simulink model "mcb_pmsm_foc_sensorless_dyno_f28379d"  (R2024b)
settings: Solver=FixedStepDiscrete  StartTime=0.0  StopTime=6  RelTol=1e-3  EnableMultiTasking=on
InitFcn:
  | mcb_pmsm_foc_sensorless_dyno_f28379d_datascript;
model workspace (MAT data in the model file):
  encoderResolution = 2000
  hallOffset = '0.5'
  indexOffset = 850
  polePairs = '4'
undefined symbols (not defined in the file or in its folder): acceleration, dataType, Down, GPTRIP1SEL, GPTRIP2SEL, inverter_motor1, inverter_motor2, PI_params_motor1, PI_params_motor2, pmsm_motor1, pmsm_motor2, PU_System_motor1, PU_System_motor2, PWM_frequency, SlidFCS_params, Speed_openLoop_PU, T_Ref_openLoop, target, Ts, Ts_motor, Ts_simulink, Ts_speed, TZ1, TZ2, Up, Vd_Ref_openLoop_PU
libraries: mcbcontrolslib x20, c2802xlib x14, simulink x8, c280xlib x7, slpidlib x5, c2837xDlib x5, mcbpositiondecoderlib x4, svdschedulerlib x3, mcbsensorlessestimatorlib x2, mcbpmsmnonlinearlib x2, autolibpmsmexterior x2, mcbplantlib x2
(part 4 of 4)

== system mcb_pmsm_foc_sensorless_dyno_f28379d/FOC Algorithm Motor 2/Enable Motor2 after a delay/Delay to start motor2 (codegen)/Disable EnMtr2TrqCtrl ==
  Enable : EnablePort  StatesWhenEnabling=reset
  Constant : Constant  Value=0  OutDataTypeStr=boolean
  Data Store Write : DataStoreWrite  DataStoreName=EnMtr2TrqCtrl  IndexOptions=Index vector (dialog)  Indices=1  OutputSizes=1
  wires:
  Constant/1 -> Data Store Write/1

== system mcb_pmsm_foc_sensorless_dyno_f28379d/FOC Algorithm Motor 2/Enable Motor2 after a delay/Delay to start motor2 (codegen)/Enable EnMtr2TrqCtrl after 2 sec delay ==
  Enable : EnablePort  StatesWhenEnabling=reset
  Add : Sum
  Constant : Constant  OutDataTypeStr=boolean
  Constant1 : Constant  Value=0  OutDataTypeStr=boolean
  Constant2 : Constant  OutDataTypeStr=uint32
  Enable EnMtr2TrqCtrl : Subsystem  TreatAsAtomicUnit=on
  Switch : Switch  Criteria=u2 > Threshold  Threshold=2*PWM_frequency  SaturateOnIntegerOverflow=off  InputSameDT=off
  Unit Delay : UnitDelay  SampleTime=-1  HasFrameUpgradeWarning=on
  wires:
  Constant1/1 -> Switch/3
  Constant/1 -> Switch/1
  Constant2/1 -> Add/1
  Add/1 -> Unit Delay/1, Switch/2
  Unit Delay/1 -> Add/2
  Switch/1 -> Enable EnMtr2TrqCtrl/Enable

== system mcb_pmsm_foc_sensorless_dyno_f28379d/FOC Algorithm Motor 2/Enable Motor2 after a delay/Delay to start motor2 (sim)/Delay 0.5 sec ==
  Enable : EnablePort  StatesWhenEnabling=reset
  Add : Sum
  Constant : Constant  OutDataTypeStr=boolean
  Constant1 : Constant  Value=0  OutDataTypeStr=boolean
  Constant2 : Constant  OutDataTypeStr=uint32
  Switch : Switch  Criteria=u2 > Threshold  Threshold=PWM_frequency/2  SaturateOnIntegerOverflow=off  InputSameDT=off
  Unit Delay : UnitDelay  SampleTime=-1  HasFrameUpgradeWarning=on
  Out1 : Outport
  wires:
  Constant1/1 -> Switch/3
  Constant/1 -> Switch/1
  Constant2/1 -> Add/1
  Add/1 -> Unit Delay/1, Switch/2
  Unit Delay/1 -> Add/2
  Switch/1 -> Out1/1

== system mcb_pmsm_foc_sensorless_dyno_f28379d/FOC Algorithm Motor 2/Enable Motor2 after a delay/Delay to start motor2 (sim)/Enabled Subsystem ==
  Enable : EnablePort
  Constant : Constant  OutDataTypeStr=boolean
  Data Store Write : DataStoreWrite  DataStoreName=EnMtr2TrqCtrl  IndexOptions=Index vector (dialog)  Indices=1  OutputSizes=1
  wires:
  Constant/1 -> Data Store Write/1

== system mcb_pmsm_foc_sensorless_dyno_f28379d/FOC Algorithm Motor 2/Enable Motor2 after a delay/Delay to start motor2 (sim)/Enabled Subsystem2 ==
  Enable : EnablePort
  Constant : Constant  Value=0  OutDataTypeStr=boolean
  Data Store Write : DataStoreWrite  DataStoreName=EnMtr2TrqCtrl  IndexOptions=Index vector (dialog)  Indices=1  OutputSizes=1
  wires:
  Constant/1 -> Data Store Write/1

== system mcb_pmsm_foc_sensorless_dyno_f28379d/FOC Algorithm Motor 2/Input Scaling/Calculate Phase Currents/Data_Type ==
  In1 : Inport
  Data_Type_Fixed_Point : Subsystem  VariantControl=~isequal(dataType,'single')
  Data_Type_Float : Subsystem  VariantControl=isequal(dataType,'single')
  Iab_meas_PU : Outport

== system mcb_pmsm_foc_sensorless_dyno_f28379d/FOC Algorithm Motor 2/Input Scaling/Calculate position and speed/Flux Observer ==
  InputSignals : Inport
  Action Port : ActionPort  ActionPortLabel=case [ 1 ]:
  DC component removal : Subsystem
  Data Store Read1 : DataStoreRead  DataStoreName=Enable  IndexOptions=Index vector (dialog)  Indices=1  OutputSizes=1
  Demux2 : Demux
  Flux Observer : mcbpositiondecoderlib/Flux Observer  MotorSelection=PMSM  DataTypeSelect=off  BlockInputUnit=Per-unit  PerUnitVoltage=PU_System_motor2.V_base  PerUnitCurrent=PU_System_motor2.I_base  PositionSelect=on  FluxSelect=off  TorqueSelect=off  PolePairs=4  StatorResistance=pmsm_motor2.Rs  StatorDAxisInductance=pmsm_motor2.Ld  StatorLeakageInductance=0.0068  RotorLeakageInductance=0.0068  MagnetizingInductance=0.0300  CutoffFreq=3.1863  BlockSampleTime=Ts  ParameterBusInput=off  PositionUnit=Per-unit  PositionDatatype=dataType  FluxUnit=Weber  PerUnitFlux=0.1  FluxDatatype=single  TorqueUnit=Nm  PerUnitTorque=100  TorqueDatatype=single  DataType=0
  IIR Filter : mcbcontrolslib/IIR Filter  VariantControl=Low Pass Filter  VariantSelect=Low-pass  FilterConstantInputType=Specify via dialog  Filter_constant=0.01  advancedSettings=off  Ts=50e-6  cutOff_freq=32.1525
  Logical Operator : Logic  Operator=NOT  IconShape=distinctive  AllPortsSameDT=off  OutDataTypeStr=boolean
  Mux2 : Mux  Inputs=2
  Speed Measurement : mcbpositiondecoderlib/Speed Measurement  PositionUnit=Per unit  PositionScalingDatatype=uint32  SpeedCalculationMode=Time interval for speed calculation  SampleTimeAsync=Ts  MaximumApplicationSpeed=60000  SpeedResolution=5e-6  DelayLength=10  MaximumMeasurableSpeed=59999  MeasurableSpeedResolution=2.794e-05  SpeedUnit=Per unit based on dialog  PerUnitSpeed=PU_System_motor2.N_base  SpeedDataType=dataType
  elect2mech : Gain  Gain=1/pmsm_motor2.p  RndMeth=Simplest  OutDataTypeStr=Inherit: Same as input
  Position/Speed : Outport
  wires:
  InputSignals/1 -> DC component removal/1(SigIN)
  Demux2/1 -> Flux Observer/1
  Demux2/2 -> Flux Observer/2
  Mux2/1 -> Position/Speed/1
  Speed Measurement/1 -> IIR Filter/1
  elect2mech/1 -> Mux2/2
  Demux2/3 -> Flux Observer/3  "Ialpha"
  Demux2/4 -> Flux Observer/4  "Ibeta"
  IIR Filter/1 -> elect2mech/1
  Flux Observer/1 -> Mux2/1, Speed Measurement/1
  Logical Operator/1 -> Flux Observer/5
  Data Store Read1/1 -> Logical Operator/1
  DC component removal/1(SigOUT) -> Demux2/1

== system mcb_pmsm_foc_sensorless_dyno_f28379d/FOC Algorithm Motor 2/Input Scaling/Calculate position and speed/Sliding Mode Observer ==
  InputSignals : Inport
  Action Port : ActionPort  ActionPortLabel=case [ 0 ]:
  Data Store Read1 : DataStoreRead  DataStoreName=Enable  IndexOptions=Index vector (dialog)  Indices=1  OutputSizes=1
  Demux1 : Demux
  Logical Operator : Logic  Operator=NOT  IconShape=distinctive  AllPortsSameDT=off  OutDataTypeStr=boolean
  Mux : Mux  Inputs=2
  Sliding Mode Observer : mcbsensorlessestimatorlib/Sliding Mode Observer  InputUnit=Per-unit  BlkSampleTime=Ts  StatorResistance=pmsm_motor2.Rs  StatorInductance=pmsm_motor2.Ld  MaxApplicationSpeed=pmsm_motor2.N_base  PolePairs=pmsm_motor2.p  MaxStatorVoltage=PU_System_motor2.V_base  MaxStatorCurrent=PU_System_motor2.I_base  DisturbanceObserverGain=smo_motor2.BackEmfObsGain  CurrentObserverGain=smo_motor2.CurrentObsGain  CutoffFreq=smo_motor2.CutoffFreq  PositionUnit=Per unit  PositionDataType=dataType  SpeedUnit=Per unit  PerUnitSpeed=PU_System_motor2.N_base  SpeedDataType=dataType
  Position/Speed : Outport
  wires:
  Mux/1 -> Position/Speed/1
  Demux1/1 -> Sliding Mode Observer/1
  Demux1/2 -> Sliding Mode Observer/2
  Demux1/4 -> Sliding Mode Observer/4  "Ibeta"
  Demux1/3 -> Sliding Mode Observer/3  "Ialpha"
  Sliding Mode Observer/1 -> Mux/1
  Sliding Mode Observer/2 -> Mux/2
  InputSignals/1 -> Demux1/1
  Data Store Read1/1 -> Logical Operator/1
  Logical Operator/1 -> Sliding Mode Observer/5

== system mcb_pmsm_foc_sensorless_dyno_f28379d/Hardware Init/HW_Init/HW_Init (Codegen)/Calibrate ADC offset for motor 1 current sensor ==
  note: Enable ADC offset calibration only when motor is not loaded and not rotating due to external factors
  ADC Calib Enable : Constant  Value=inverter_motor1.ADCOffsetCalibEnable  OutDataTypeStr=Inherit: Inherit via back propagation
  "Calculate ADC Offset " : Subsystem  Priority=1001  TreatAsAtomicUnit=on
  Default ADC Offset : Subsystem  Priority=1001  TreatAsAtomicUnit=on
  NOT : Logic  Operator=NOT  IconShape=distinctive  AllPortsSameDT=off  OutDataTypeStr=boolean
  wires:
  NOT/1 -> Default ADC Offset/Enable
  ADC Calib Enable/1 -> "Calculate ADC Offset "/Enable, NOT/1

== system mcb_pmsm_foc_sensorless_dyno_f28379d/Hardware Init/HW_Init/HW_Init (Codegen)/Calibrate ADC offset for motor 2 current sensor ==
  note: Enable ADC offset calibration only when motor is not loaded and not rotating due to external factors
  ADC Calib Enable : Constant  Value=inverter_motor2.ADCOffsetCalibEnable  OutDataTypeStr=Inherit: Inherit via back propagation
  Calculate ADC Offset : Subsystem  Priority=1001  TreatAsAtomicUnit=on
  Default ADC Offset : Subsystem  Priority=1001  TreatAsAtomicUnit=on
  NOT : Logic  Operator=NOT  IconShape=distinctive  AllPortsSameDT=off  OutDataTypeStr=boolean
  wires:
  ADC Calib Enable/1 -> Calculate ADC Offset/Enable, NOT/1
  NOT/1 -> Default ADC Offset/Enable

== system mcb_pmsm_foc_sensorless_dyno_f28379d/Hardware Init/HW_Init/HW_Init (Codegen)/Enable DRV8305 for motor 1 and motor 2 ==
  note: Enable DRV8305 for Motor 1
  note: Enable DRV8305 for Motor 2
  6PWM_Mode : Constant  Priority=1000  Value=0x3A16  OutDataTypeStr=uint16  SampleTime=-1
  6PWM_Mode1 : Constant  Priority=1000  Value=0x3A16  OutDataTypeStr=uint16  SampleTime=-1
  ADC_Gain_Setting : Constant  Priority=1000  Value=inverter_motor1.SPI_Gain_Setting  OutDataTypeStr=uint16  SampleTime=-1
  ADC_Gain_Setting1 : Constant  Priority=1000  Value=inverter_motor2.SPI_Gain_Setting  OutDataTypeStr=uint16  SampleTime=-1
  Bottom DRV8305 EN : c2837xDlib/Digital Output  GPIO_Number=GPIO24~GPIO31  GPIO_Bit0=off  GPIO_BIT0_Toggle=off  GPIO_Bit1=off  GPIO_BIT1_Toggle=off  GPIO_Bit2=on  GPIO_BIT2_Toggle=off  GPIO_Bit3=off  GPIO_BIT3_Toggle=off  GPIO_Bit4=off  GPIO_BIT4_Toggle=off  GPIO_Bit5=off  GPIO_BIT5_Toggle=off  GPIO_Bit6=off  GPIO_BIT6_Toggle=off  GPIO_Bit7=off  GPIO_BIT7_Toggle=off
  DRV830x Enable : Constant  OutDataTypeStr=uint16  SampleTime=-1
  DRV830x Enable3 : Constant  OutDataTypeStr=uint16  SampleTime=-1
  Digital Output : c2837xDlib/Digital Output  Priority=10  GPIO_Number=GPIO120~GPIO127  GPIO_Bit0=off  GPIO_BIT0_Toggle=off  GPIO_Bit1=off  GPIO_BIT1_Toggle=off  GPIO_Bit2=off  GPIO_BIT2_Toggle=off  GPIO_Bit3=off  GPIO_BIT3_Toggle=off  GPIO_Bit4=on  GPIO_BIT4_Toggle=off  GPIO_Bit5=off  GPIO_BIT5_Toggle=off  GPIO_Bit6=off  GPIO_BIT6_Toggle=off  GPIO_Bit7=off  GPIO_BIT7_Toggle=off
  Display{,1..3} (4 alike) : Display
      settings: Format=hex (Stored Integer)
  SPI Master Transfer : c280xlib/SPI Controller Transfer  SPISelect=SPI_A  ClockPolarity=Rising_edge  ClockPhase=No_delay  SPIModule=uint32(0)  Mode=Master  BusSpeed=uint32(1000000)  FirstBitToTransfer=Most significant bit (MSB)  ClockMode=0  BlockFunction=Transfer  EnableRegisterAddress=off  RegisterAddress=0  OutputDataType=int8  OutputDataLength=1  DataBits=16  UseCustomSSPin=Provided by the SPI peripheral  ActiveLowSSPin=Active low  Pin=61
  SPI Master Transfer1 : c280xlib/SPI Controller Transfer  SPISelect=SPI_A  ClockPolarity=Rising_edge  ClockPhase=No_delay  SPIModule=uint32(0)  Mode=Master  BusSpeed=uint32(1000000)  FirstBitToTransfer=Most significant bit (MSB)  ClockMode=0  BlockFunction=Transfer  EnableRegisterAddress=off  RegisterAddress=0  OutputDataType=int8  OutputDataLength=1  DataBits=16  UseCustomSSPin=Provided by the SPI peripheral  ActiveLowSSPin=Active low  Pin=61
  SPI Master Transfer2 : c280xlib/SPI Controller Transfer  SPISelect=SPI_B  ClockPolarity=Rising_edge  ClockPhase=No_delay  SPIModule=uint32(0)  Mode=Master  BusSpeed=uint32(1000000)  FirstBitToTransfer=Most significant bit (MSB)  ClockMode=0  BlockFunction=Transfer  EnableRegisterAddress=off  RegisterAddress=0  OutputDataType=int8  OutputDataLength=1  DataBits=16  UseCustomSSPin=Provided by the SPI peripheral  ActiveLowSSPin=Active low  Pin=61
  SPI Master Transfer3 : c280xlib/SPI Controller Transfer  SPISelect=SPI_B  ClockPolarity=Rising_edge  ClockPhase=No_delay  SPIModule=uint32(0)  Mode=Master  BusSpeed=uint32(1000000)  FirstBitToTransfer=Most significant bit (MSB)  ClockMode=0  BlockFunction=Transfer  EnableRegisterAddress=off  RegisterAddress=0  OutputDataType=int8  OutputDataLength=1  DataBits=16  UseCustomSSPin=Provided by the SPI peripheral  ActiveLowSSPin=Active low  Pin=61
  wires:
  DRV830x Enable/1 -> Digital Output/1
  DRV830x Enable3/1 -> Bottom DRV8305 EN/1
  6PWM_Mode1/1 -> SPI Master Transfer2/1
  6PWM_Mode/1 -> SPI Master Transfer/1
  ADC_Gain_Setting/1 -> SPI Master Transfer1/1
  SPI Master Transfer3/1 -> Display3/1
  SPI Master Transfer2/1 -> Display2/1
  SPI Master Transfer1/1 -> Display1/1
  SPI Master Transfer/1 -> Display/1
  ADC_Gain_Setting1/1 -> SPI Master Transfer3/1

== system mcb_pmsm_foc_sensorless_dyno_f28379d/Serial Receive/Parse SCI Rx/Data_Conditioning_Rx/Data_Type_Fixed_Point ==
  Rx : Inport
  Data Type Conversion1 : DataTypeConversion  OutDataTypeStr=dataType  RndMeth=Simplest  SaturateOnIntegerOverflow=off
  Data Type Conversion2 : DataTypeConversion  OutDataTypeStr=fixdt(1,32,28)  ConvertRealWorld=Stored Integer (SI)  RndMeth=Simplest  SaturateOnIntegerOverflow=off
  Data Type Conversion3 : DataTypeConversion  OutDataTypeStr=uint16  RndMeth=Simplest  SaturateOnIntegerOverflow=off
  Data Type Conversion4 : DataTypeConversion  OutDataTypeStr=dataType  RndMeth=Simplest  SaturateOnIntegerOverflow=off
  Data Type Conversion5 : DataTypeConversion  OutDataTypeStr=fixdt(1,32,28)  ConvertRealWorld=Stored Integer (SI)  RndMeth=Simplest  SaturateOnIntegerOverflow=off
  Demux : Demux  Outputs=3
  Desired Speed : Outport
  Out2 : Outport  Port=2
  Desired torque : Outport  Port=3
  wires:
  Rx/1 -> Demux/1
  Data Type Conversion1/1 -> Desired Speed/1
  Data Type Conversion2/1 -> Data Type Conversion1/1
  Demux/1 -> Data Type Conversion2/1
  Demux/2 -> Data Type Conversion3/1
  Data Type Conversion3/1 -> Out2/1
  Demux/3 -> Data Type Conversion5/1
  Data Type Conversion5/1 -> Data Type Conversion4/1
  Data Type Conversion4/1 -> Desired torque/1

== system mcb_pmsm_foc_sensorless_dyno_f28379d/Serial Receive/Parse SCI Rx/Data_Conditioning_Rx/Data_Type_Float ==
  Rx : Inport
  Data Type Conversion2 : DataTypeConversion  OutDataTypeStr=uint16  RndMeth=Simplest  SaturateOnIntegerOverflow=off
  Demux : Demux  Outputs=3
  Desired Speed : Outport
  Out2 : Outport  Port=2
  Desired torque : Outport  Port=3
  wires:
  Rx/1 -> Demux/1
  Demux/1 -> Desired Speed/1
  Data Type Conversion2/1 -> Out2/1
  Demux/2 -> Data Type Conversion2/1
  Demux/3 -> Desired torque/1

== system mcb_pmsm_foc_sensorless_dyno_f28379d/Serial Receive/Serial Receive/Serial Rx/Data_Type_Fixed_Point ==
  SCI Receive : c280xlib/SCI Receive  sciModule=A  dataHead=''  headerCheckMaxCount=16  dataTail=''  dataType=uint32  dataLenOptions=Length via dialog  dataDim=3  maxDataLength=1  initValue=0  errOption=Output the last received value  errValue=0  sampleTime=-1  blockingMode=on  timeOut=0.00875  outputStatus=off
  Rx : Outport
  wires:
  SCI Receive/1 -> Rx/1

== system mcb_pmsm_foc_sensorless_dyno_f28379d/Serial Receive/Serial Receive/Serial Rx/Data_Type_Float ==
  SCI Receive : c280xlib/SCI Receive  sciModule=A  dataHead=''  headerCheckMaxCount=16  dataTail=''  dataType=single  dataLenOptions=Length via dialog  dataDim=3  maxDataLength=1  initValue=0  errOption=Output the last received value  errValue=0  sampleTime=-1  blockingMode=on  timeOut=0.00875  outputStatus=off
  Rx : Outport
  wires:
  SCI Receive/1 -> Rx/1

== system mcb_pmsm_foc_sensorless_dyno_f28379d/Serial Receive/Signal Packing/Data_Conditioning_Tx/Data_Type_Fixed_Point ==
  In1 : Inport
  In2 : Inport  Port=2
  In3 : Inport  Port=3
  Data Type Conversion : DataTypeConversion  OutDataTypeStr=fixdt(1,32,28)  RndMeth=Simplest  SaturateOnIntegerOverflow=off
  Data Type Conversion1 : DataTypeConversion  OutDataTypeStr=uint32  RndMeth=Simplest  SaturateOnIntegerOverflow=off
  Data Type Conversion2 : DataTypeConversion  OutDataTypeStr=fixdt(1,32,28)  RndMeth=Simplest  SaturateOnIntegerOverflow=off
  Data Type Conversion3 : DataTypeConversion  OutDataTypeStr=uint32  ConvertRealWorld=Stored Integer (SI)  RndMeth=Simplest  SaturateOnIntegerOverflow=off
  Data Type Conversion4 : DataTypeConversion  OutDataTypeStr=uint32  ConvertRealWorld=Stored Integer (SI)  RndMeth=Simplest  SaturateOnIntegerOverflow=off
  Mux : Mux  Inputs=3
  Data : Outport
  wires:
  In1/1 -> Data Type Conversion/1
  Data Type Conversion3/1 -> Mux/1
  Data Type Conversion/1 -> Data Type Conversion3/1
  In2/1 -> Data Type Conversion1/1
  Data Type Conversion1/1 -> Mux/2
  Mux/1 -> Data/1
  Data Type Conversion2/1 -> Data Type Conversion4/1
  Data Type Conversion4/1 -> Mux/3
  In3/1 -> Data Type Conversion2/1

== system mcb_pmsm_foc_sensorless_dyno_f28379d/Serial Receive/Signal Packing/Data_Conditioning_Tx/Data_Type_Float ==
  In1 : Inport
  In2 : Inport  Port=2
  In3 : Inport  Port=3
  Data Type Conversion2 : DataTypeConversion  OutDataTypeStr=single  RndMeth=Simplest  SaturateOnIntegerOverflow=off
  Mux : Mux  Inputs=3
  Data : Outport
  wires:
  In1/1 -> Mux/1
  Mux/1 -> Data/1
  In2/1 -> Data Type Conversion2/1
  Data Type Conversion2/1 -> Mux/2
  In3/1 -> Mux/3

== system mcb_pmsm_foc_sensorless_dyno_f28379d/FOC Algorithm Motor 1/Input Scaling/Calculate Phase Currents/Data_Type/Data_Type_Fixed_Point ==
  In1 : Inport
  Data Type Conversion : DataTypeConversion  OutDataTypeStr=fixdt(1,32,17)  ConvertRealWorld=Stored Integer (SI)  RndMeth=Simplest  SaturateOnIntegerOverflow=off
  Data Type Conversion1 : DataTypeConversion  OutDataTypeStr=dataType  RndMeth=Simplest  SaturateOnIntegerOverflow=off
  Q17 per unit conversion : ArithShift  BitShiftNumber=-6
  Iab_meas_PU : Outport
  wires:
  In1/1 -> Q17 per unit conversion/1
  Data Type Conversion1/1 -> Iab_meas_PU/1
  Data Type Conversion/1 -> Data Type Conversion1/1
  Q17 per unit conversion/1 -> Data Type Conversion/1

== system mcb_pmsm_foc_sensorless_dyno_f28379d/FOC Algorithm Motor 1/Input Scaling/Calculate Phase Currents/Data_Type/Data_Type_Float ==
  In1 : Inport
  Get ADC Voltage : Gain  Gain=target.ADC_Vref /target.ADC_MaxCount  OutDataTypeStr=dataType  RndMeth=Simplest
  Get Currents : Gain  Gain=1/inverter_motor1.ISenseVoltPerAmp  RndMeth=Simplest  OutDataTypeStr=Inherit: Same as input
  PU_Conversion : Gain  Gain=1/PU_System_motor1.I_base  RndMeth=Simplest  OutDataTypeStr=Inherit: Same as input
  Iab_meas_PU : Outport
  wires:
  Get ADC Voltage/1 -> Get Currents/1
  Get Currents/1 -> PU_Conversion/1
  PU_Conversion/1 -> Iab_meas_PU/1
  In1/1 -> Get ADC Voltage/1

== system mcb_pmsm_foc_sensorless_dyno_f28379d/FOC Algorithm Motor 1/Input Scaling/Calculate position and speed/Flux Observer/DC component removal ==
  SigIN : Inport
  IIR Filter : mcbcontrolslib/IIR Filter  VariantControl=Low Pass Filter  VariantSelect=Low-pass  FilterConstantInputType=Specify via dialog  Filter_constant=0.005*(Ts/50e-6)  advancedSettings=off  Ts=50e-6  cutOff_freq=15.9955
  Sum6 : Sum  Inputs=|+-  RndMeth=Simplest  OutDataTypeStr=Inherit: Same as first input
  SigOUT : Outport
  wires:
  IIR Filter/1 -> Sum6/2
  SigIN/1 -> IIR Filter/1, Sum6/1
  Sum6/1 -> SigOUT/1

== system mcb_pmsm_foc_sensorless_dyno_f28379d/FOC Algorithm Motor 2/Enable Motor2 after a delay/Delay to start motor2 (codegen)/Enable EnMtr2TrqCtrl after 2 sec delay/Enable EnMtr2TrqCtrl ==
  Enable : EnablePort  StatesWhenEnabling=reset
  Constant : Constant  OutDataTypeStr=boolean
  Data Store Write : DataStoreWrite  DataStoreName=EnMtr2TrqCtrl  IndexOptions=Index vector (dialog)  Indices=1  OutputSizes=1
  wires:
  Constant/1 -> Data Store Write/1

== system mcb_pmsm_foc_sensorless_dyno_f28379d/FOC Algorithm Motor 2/Input Scaling/Calculate Phase Currents/Data_Type/Data_Type_Fixed_Point ==
  In1 : Inport
  Data Type Conversion : DataTypeConversion  OutDataTypeStr=fixdt(1,32,17)  ConvertRealWorld=Stored Integer (SI)  RndMeth=Simplest  SaturateOnIntegerOverflow=off
  Data Type Conversion1 : DataTypeConversion  OutDataTypeStr=dataType  RndMeth=Simplest  SaturateOnIntegerOverflow=off
  Q17 per unit conversion : ArithShift  BitShiftNumber=-6
  Iab_meas_PU : Outport
  wires:
  Q17 per unit conversion/1 -> Data Type Conversion/1
  Data Type Conversion/1 -> Data Type Conversion1/1
  Data Type Conversion1/1 -> Iab_meas_PU/1
  In1/1 -> Q17 per unit conversion/1

== system mcb_pmsm_foc_sensorless_dyno_f28379d/FOC Algorithm Motor 2/Input Scaling/Calculate Phase Currents/Data_Type/Data_Type_Float ==
  In1 : Inport
  Get ADC Voltage : Gain  Gain=target.ADC_Vref /target.ADC_MaxCount  OutDataTypeStr=dataType  RndMeth=Simplest
  Get Currents : Gain  Gain=1/inverter_motor2.ISenseVoltPerAmp  RndMeth=Simplest  OutDataTypeStr=Inherit: Same as input
  PU_Conversion : Gain  Gain=1/PU_System_motor2.I_base  RndMeth=Simplest  OutDataTypeStr=Inherit: Same as input
  Iab_meas_PU : Outport
  wires:
  Get ADC Voltage/1 -> Get Currents/1
  Get Currents/1 -> PU_Conversion/1
  PU_Conversion/1 -> Iab_meas_PU/1
  In1/1 -> Get ADC Voltage/1

== system mcb_pmsm_foc_sensorless_dyno_f28379d/FOC Algorithm Motor 2/Input Scaling/Calculate position and speed/Flux Observer/DC component removal ==
  SigIN : Inport
  IIR Filter : mcbcontrolslib/IIR Filter  VariantControl=Low Pass Filter  VariantSelect=Low-pass  FilterConstantInputType=Specify via dialog  Filter_constant=0.005*(Ts/50e-6)  advancedSettings=off  Ts=50e-6  cutOff_freq=15.9955
  Sum6 : Sum  Inputs=|+-  RndMeth=Simplest  OutDataTypeStr=Inherit: Same as first input
  SigOUT : Outport
  wires:
  IIR Filter/1 -> Sum6/2
  SigIN/1 -> IIR Filter/1, Sum6/1
  Sum6/1 -> SigOUT/1

== system mcb_pmsm_foc_sensorless_dyno_f28379d/Hardware Init/HW_Init/HW_Init (Codegen)/Calibrate ADC offset for motor 1 current sensor/Calculate ADC Offset  ==
  Enable : EnablePort
  Constant : Constant  Value=8
  Constant1 : Constant  Value=inverter_motor1.CtSensOffsetMax  OutDataTypeStr=Inherit: Inherit via back propagation
  Constant2 : Constant  Value=inverter_motor1.CtSensOffsetMin  OutDataTypeStr=Inherit: Inherit via back propagation
  Divide : Product  Inputs=*/  OutDataTypeStr=uint16
  Divide1 : Product  Inputs=*/  OutDataTypeStr=uint16
  For Iterator Subsystem : Subsystem  TreatAsAtomicUnit=on
  If : If  NumInputs=3  IfExpression=u1 > u3 & u1 < u2
  If Action Subsystem : Subsystem  TreatAsAtomicUnit=on
  If Action Subsystem1 : Subsystem  TreatAsAtomicUnit=on
  If Action Subsystem2 : Subsystem  TreatAsAtomicUnit=on
  If Action Subsystem3 : Subsystem  TreatAsAtomicUnit=on
  If1 : If  NumInputs=3  IfExpression=u1 > u3 & u1 < u2
  wires:
  For Iterator Subsystem/2(Out2) -> Divide1/1
  Divide/1 -> If Action Subsystem/1(In1), If/1
  For Iterator Subsystem/1(Out1) -> Divide/1
  Constant/1 -> Divide/2, Divide1/2
  Divide1/1 -> If1/1, If Action Subsystem2/1(In1)
  If/1 -> If Action Subsystem/Action
  If/2 -> If Action Subsystem1/Action
  If1/1 -> If Action Subsystem2/Action
  If1/2 -> If Action Subsystem3/Action
  Constant1/1 -> If/2, If1/2
  Constant2/1 -> If/3, If1/3

== system mcb_pmsm_foc_sensorless_dyno_f28379d/Hardware Init/HW_Init/HW_Init (Codegen)/Calibrate ADC offset for motor 1 current sensor/Default ADC Offset ==
  Enable : EnablePort
  Constant : Constant  Value=inverter_motor1.CtSensAOffset  OutDataTypeStr=Inherit: Inherit via back propagation
  Constant1 : Constant  Value=inverter_motor1.CtSensBOffset  OutDataTypeStr=Inherit: Inherit via back propagation
  Data Store Write1 : DataStoreWrite  DataStoreName=IaOffset_motor1  IndexOptions=Index vector (dialog)  Indices=1  OutputSizes=1
  Data Store Write2 : DataStoreWrite  DataStoreName=IbOffset_motor1  IndexOptions=Index vector (dialog)  Indices=1  OutputSizes=1
  wires:
  Constant/1 -> Data Store Write1/1
  Constant1/1 -> Data Store Write2/1

== system mcb_pmsm_foc_sensorless_dyno_f28379d/Hardware Init/HW_Init/HW_Init (Codegen)/Calibrate ADC offset for motor 2 current sensor/Calculate ADC Offset ==
  Enable : EnablePort
  Constant1 : Constant  Value=8
  Constant2 : Constant  Value=inverter_motor2.CtSensOffsetMax  OutDataTypeStr=Inherit: Inherit via back propagation
  Constant3 : Constant  Value=inverter_motor2.CtSensOffsetMin  OutDataTypeStr=Inherit: Inherit via back propagation
  Divide2 : Product  Inputs=*/  OutDataTypeStr=uint16
  Divide3 : Product  Inputs=*/  OutDataTypeStr=uint16
  For Iterator Subsystem : Subsystem  TreatAsAtomicUnit=on
  If Action Subsystem4 : Subsystem  TreatAsAtomicUnit=on
  If Action Subsystem5 : Subsystem  TreatAsAtomicUnit=on
  If Action Subsystem6 : Subsystem  TreatAsAtomicUnit=on
  If Action Subsystem7 : Subsystem  TreatAsAtomicUnit=on
  If2 : If  NumInputs=3  IfExpression=u1 > u3 & u1 < u2
  If3 : If  NumInputs=3  IfExpression=u1 > u3 & u1 < u2
  wires:
  For Iterator Subsystem/2(Out4) -> Divide3/1
  Divide2/1 -> If2/1, If Action Subsystem4/1(In1)
  For Iterator Subsystem/1(Out3) -> Divide2/1
  Constant1/1 -> Divide2/2, Divide3/2
  Divide3/1 -> If3/1, If Action Subsystem6/1(In1)
  If2/1 -> If Action Subsystem4/Action
  If2/2 -> If Action Subsystem5/Action
  If3/1 -> If Action Subsystem6/Action
  If3/2 -> If Action Subsystem7/Action
  Constant2/1 -> If2/2, If3/2
  Constant3/1 -> If2/3, If3/3

== system mcb_pmsm_foc_sensorless_dyno_f28379d/Hardware Init/HW_Init/HW_Init (Codegen)/Calibrate ADC offset for motor 2 current sensor/Default ADC Offset ==
  Enable : EnablePort
  Constant2 : Constant  Value=inverter_motor2.CtSensAOffset  OutDataTypeStr=Inherit: Inherit via back propagation
  Constant3 : Constant  Value=inverter_motor2.CtSensBOffset  OutDataTypeStr=Inherit: Inherit via back propagation
  Data Store Write3 : DataStoreWrite  DataStoreName=IaOffset_motor2  IndexOptions=Index vector (dialog)  Indices=1  OutputSizes=1
  Data Store Write4 : DataStoreWrite  DataStoreName=IbOffset_motor2  IndexOptions=Index vector (dialog)  Indices=1  OutputSizes=1
  wires:
  Constant2/1 -> Data Store Write3/1
  Constant3/1 -> Data Store Write4/1

== system mcb_pmsm_foc_sensorless_dyno_f28379d/Hardware Init/HW_Init/HW_Init (Codegen)/Calibrate ADC offset for motor 1 current sensor/Calculate ADC Offset /For Iterator Subsystem ==
  ADC_A_IN0 : c2802xlib/ADC  Priority=20  blkParamProc=C2000_Type4  ADCModule=C  samplingMode=Single sample mode  ADCResolution=12-bit (Single-ended input)  useSOC1=SOC2  useSOC2=SOC0_SOC1  SOCAcquisitionWindow=15  SOCTriggerSource=Software  SOCInterruptTrigger=No ADCINT  Ts=-1  dType=uint16  postInterrupt=off  interruptSel=ADCINT1  ADCINTContinuous=on  endma=off  chdma=1  conv1=ADCINA0  conv2=ADCINA0 and ADCINB0  conv1_Type4=ADCIN2  conv2_Type4=ADCIN0 and ADCIN1
  ADC_B_IN0 : c2802xlib/ADC  Priority=20  blkParamProc=C2000_Type4  ADCModule=B  samplingMode=Single sample mode  ADCResolution=12-bit (Single-ended input)  useSOC1=SOC2  useSOC2=SOC0_SOC1  SOCAcquisitionWindow=15  SOCTriggerSource=Software  SOCInterruptTrigger=No ADCINT  Ts=-1  dType=uint16  postInterrupt=off  interruptSel=ADCINT1  ADCINTContinuous=on  endma=off  chdma=1  conv1=ADCINA0  conv2=ADCINA0 and ADCINB0  conv1_Type4=ADCIN2  conv2_Type4=ADCIN0 and ADCIN1
  For Iterator : ForIterator  IterationLimit=16  IterationVariableDataType=uint16
  If : If  IfExpression=u1 > 8  ShowElse=off
  If Action Subsystem : Subsystem  TreatAsAtomicUnit=on
  Out1 : Outport
  Out2 : Outport  Port=2
  wires:
  For Iterator/1 -> If/1
  ADC_A_IN0/1 -> If Action Subsystem/1(In1)
  ADC_B_IN0/1 -> If Action Subsystem/2(In2)
  If Action Subsystem/1(Out1) -> Out1/1
  If Action Subsystem/2(Out2) -> Out2/1
  If/1 -> If Action Subsystem/Action

== system mcb_pmsm_foc_sensorless_dyno_f28379d/Hardware Init/HW_Init/HW_Init (Codegen)/Calibrate ADC offset for motor 1 current sensor/Calculate ADC Offset /If Action Subsystem ==
  In1 : Inport
  Action Port : ActionPort  ActionPortLabel=if(u1 > u3 & u1 < u2)
  Data Store Write1 : DataStoreWrite  DataStoreName=IaOffset_motor1  IndexOptions=Index vector (dialog)  Indices=1  OutputSizes=1
  wires:
  In1/1 -> Data Store Write1/1

== system mcb_pmsm_foc_sensorless_dyno_f28379d/Hardware Init/HW_Init/HW_Init (Codegen)/Calibrate ADC offset for motor 1 current sensor/Calculate ADC Offset /If Action Subsystem1 ==
  Action Port : ActionPort  ActionPortLabel=else
  Constant : Constant  Value=inverter_motor1.CtSensAOffset  OutDataTypeStr=Inherit: Inherit via back propagation
  Data Store Write1 : DataStoreWrite  DataStoreName=IaOffset_motor1  IndexOptions=Index vector (dialog)  Indices=1  OutputSizes=1
  wires:
  Constant/1 -> Data Store Write1/1

== system mcb_pmsm_foc_sensorless_dyno_f28379d/Hardware Init/HW_Init/HW_Init (Codegen)/Calibrate ADC offset for motor 1 current sensor/Calculate ADC Offset /If Action Subsystem2 ==
  In1 : Inport
  Action Port : ActionPort  ActionPortLabel=if(u1 > u3 & u1 < u2)
  Data Store Write2 : DataStoreWrite  DataStoreName=IbOffset_motor1  IndexOptions=Index vector (dialog)  Indices=1  OutputSizes=1
  wires:
  In1/1 -> Data Store Write2/1

== system mcb_pmsm_foc_sensorless_dyno_f28379d/Hardware Init/HW_Init/HW_Init (Codegen)/Calibrate ADC offset for motor 1 current sensor/Calculate ADC Offset /If Action Subsystem3 ==
  Action Port : ActionPort  ActionPortLabel=else
  Constant1 : Constant  Value=inverter_motor1.CtSensBOffset  OutDataTypeStr=Inherit: Inherit via back propagation
  Data Store Write2 : DataStoreWrite  DataStoreName=IbOffset_motor1  IndexOptions=Index vector (dialog)  Indices=1  OutputSizes=1
  wires:
  Constant1/1 -> Data Store Write2/1

== system mcb_pmsm_foc_sensorless_dyno_f28379d/Hardware Init/HW_Init/HW_Init (Codegen)/Calibrate ADC offset for motor 2 current sensor/Calculate ADC Offset/For Iterator Subsystem ==
  ADC_A_IN1 : c2802xlib/ADC  Priority=20  blkParamProc=C2000_Type4  ADCModule=C  samplingMode=Single sample mode  ADCResolution=12-bit (Single-ended input)  useSOC1=SOC3  useSOC2=SOC0_SOC1  SOCAcquisitionWindow=15  SOCTriggerSource=Software  SOCInterruptTrigger=No ADCINT  Ts=-1  dType=uint16  postInterrupt=off  interruptSel=ADCINT1  ADCINTContinuous=on  endma=off  chdma=1  conv1=ADCINA0  conv2=ADCINA0 and ADCINB0  conv1_Type4=ADCIN4  conv2_Type4=ADCIN0 and ADCIN1
  ADC_B_IN1 : c2802xlib/ADC  Priority=20  blkParamProc=C2000_Type4  ADCModule=B  samplingMode=Single sample mode  ADCResolution=12-bit (Single-ended input)  useSOC1=SOC3  useSOC2=SOC0_SOC1  SOCAcquisitionWindow=15  SOCTriggerSource=Software  SOCInterruptTrigger=No ADCINT  Ts=-1  dType=uint16  postInterrupt=off  interruptSel=ADCINT1  ADCINTContinuous=on  endma=off  chdma=1  conv1=ADCINA0  conv2=ADCINA0 and ADCINB0  conv1_Type4=ADCIN4  conv2_Type4=ADCIN0 and ADCIN1
  For Iterator : ForIterator  IterationLimit=16  IterationVariableDataType=uint16
  If Action Subsystem1 : Subsystem  TreatAsAtomicUnit=on
  If1 : If  IfExpression=u1 > 8  ShowElse=off
  Out3 : Outport
  Out4 : Outport  Port=2
  wires:
  If1/1 -> If Action Subsystem1/Action
  If Action Subsystem1/2(Out2) -> Out4/1
  If Action Subsystem1/1(Out1) -> Out3/1
  ADC_B_IN1/1 -> If Action Subsystem1/2(In2)
  ADC_A_IN1/1 -> If Action Subsystem1/1(In1)
  For Iterator/1 -> If1/1

== system mcb_pmsm_foc_sensorless_dyno_f28379d/Hardware Init/HW_Init/HW_Init (Codegen)/Calibrate ADC offset for motor 2 current sensor/Calculate ADC Offset/If Action Subsystem4 ==
  In1 : Inport
  Action Port : ActionPort  ActionPortLabel=if(u1 > u3 & u1 < u2)
  Data Store Write1 : DataStoreWrite  DataStoreName=IaOffset_motor2  IndexOptions=Index vector (dialog)  Indices=1  OutputSizes=1
  wires:
  In1/1 -> Data Store Write1/1

== system mcb_pmsm_foc_sensorless_dyno_f28379d/Hardware Init/HW_Init/HW_Init (Codegen)/Calibrate ADC offset for motor 2 current sensor/Calculate ADC Offset/If Action Subsystem5 ==
  Action Port : ActionPort  ActionPortLabel=else
  Constant : Constant  Value=inverter_motor2.CtSensAOffset  OutDataTypeStr=Inherit: Inherit via back propagation
  Data Store Write1 : DataStoreWrite  DataStoreName=IaOffset_motor2  IndexOptions=Index vector (dialog)  Indices=1  OutputSizes=1
  wires:
  Constant/1 -> Data Store Write1/1

== system mcb_pmsm_foc_sensorless_dyno_f28379d/Hardware Init/HW_Init/HW_Init (Codegen)/Calibrate ADC offset for motor 2 current sensor/Calculate ADC Offset/If Action Subsystem6 ==
  In1 : Inport
  Action Port : ActionPort  ActionPortLabel=if(u1 > u3 & u1 < u2)
  Data Store Write2 : DataStoreWrite  DataStoreName=IbOffset_motor2  IndexOptions=Index vector (dialog)  Indices=1  OutputSizes=1
  wires:
  In1/1 -> Data Store Write2/1

== system mcb_pmsm_foc_sensorless_dyno_f28379d/Hardware Init/HW_Init/HW_Init (Codegen)/Calibrate ADC offset for motor 2 current sensor/Calculate ADC Offset/If Action Subsystem7 ==
  Action Port : ActionPort  ActionPortLabel=else
  Constant1 : Constant  Value=inverter_motor2.CtSensBOffset  OutDataTypeStr=Inherit: Inherit via back propagation
  Data Store Write2 : DataStoreWrite  DataStoreName=IbOffset_motor2  IndexOptions=Index vector (dialog)  Indices=1  OutputSizes=1
  wires:
  Constant1/1 -> Data Store Write2/1

== system mcb_pmsm_foc_sensorless_dyno_f28379d/Hardware Init/HW_Init/HW_Init (Codegen)/Calibrate ADC offset for motor 1 current sensor/Calculate ADC Offset /For Iterator Subsystem/If Action Subsystem ==
  In1 : Inport
  In2 : Inport  Port=2
  Action Port : ActionPort  ActionPortLabel=if(u1 > 8)
  Memory : Memory  InheritSampleTime=on
  Memory1 : Memory  InheritSampleTime=on
  Sum : Sum
  Sum1 : Sum
  Out1 : Outport
  Out2 : Outport  Port=2
  wires:
  In1/1 -> Sum/1
  Sum/1 -> Out1/1, Memory/1
  In2/1 -> Sum1/1
  Memory/1 -> Sum/2
  Sum1/1 -> Out2/1, Memory1/1
  Memory1/1 -> Sum1/2

== system mcb_pmsm_foc_sensorless_dyno_f28379d/Hardware Init/HW_Init/HW_Init (Codegen)/Calibrate ADC offset for motor 2 current sensor/Calculate ADC Offset/For Iterator Subsystem/If Action Subsystem1 ==
  In1 : Inport
  In2 : Inport  Port=2
  Action Port : ActionPort  ActionPortLabel=if(u1 > 8)
  Memory : Memory  InheritSampleTime=on
  Memory1 : Memory  InheritSampleTime=on
  Sum : Sum
  Sum1 : Sum
  Out1 : Outport
  Out2 : Outport  Port=2
  wires:
  In1/1 -> Sum/1
  Sum/1 -> Out1/1, Memory/1
  In2/1 -> Sum1/1
  Memory/1 -> Sum/2
  Sum1/1 -> Out2/1, Memory1/1
  Memory1/1 -> Sum1/2

== matlab function mcb_pmsm_foc_sensorless_dyno_f28379d/Speed Control/Subsystem/MATLAB Function2 ==
  data: Iq_ref output; sw output; params input; we input; we_past input; we_past_1 input; w_ref input; w_ref_past input; w_ref_past_1 input; sw_past input
function [Iq_ref,sw]  = DT_slid_speed(params,we,we_past,we_past_1,w_ref,w_ref_past,w_ref_past_1,sw_past)

lam1 = params(1);
lam2 = params(2);
ar = params(3);
rr = params(4);
Tc = params(5);
B = params(6);
J = params(7);
Kt = params(8);

err = we - w_ref;
err_past = we_past - w_ref_past;
err_past_1 = we_past_1 - w_ref_past_1;

% c1 = -(lam1+lam2);
% c2 = lam1*lam2;

%sw = err + c1*err_past + c2*err_past_1;
a2 = 1-lam2;
sw = a2*sw_past + err - (1-lam1*Tc)*err_past + lam2*sw_past;
sigma = sw - a2*sw_past;

%T_eq = B*we - (J/Tc)*(err*(1 + c1) + c2*err_past);
T_eq = B*we - J*(lam1*err + (lam2/Tc)*sw);
T_n = single(0);
if abs(sigma)> rr*Tc
    T_n = (ar*(J/Tc))*(abs(sigma)-(rr*Tc));
else
    if abs(sigma)<= rr*Tc
        T_n = single(0);
    end
end

Te = T_eq + T_n;

Iq_ref = Te/Kt;

== matlab function mcb_pmsm_foc_sensorless_dyno_f28379d/FOC Algorithm Motor 1/Closed Loop/Current_Controllers/Subsystem/MATLAB Function ==
  data: params input; ud output; we input; id input; iq input; id_past input; iq_past input; id_ref input; iq_ref input; id_ref_past input; iq_ref_past input; uq output; s_d output; s_q output
function [ud,uq,s_d,s_q] = DTslid(params,we,id,iq,id_past,iq_past,id_ref,iq_ref,id_ref_past,iq_ref_past)

lamd = params(1);
lamq = params(2);
ad = params(3);
aq = params(4);
rd = params(5);
rq = params(6);
Tc = params(7);
R = params(8);
Ld = params(9);
Lq = params(10);
lam0 = params(11);

err_d = id - id_ref;
err_q = iq - iq_ref;

err_d_past = id_past - id_ref_past;
err_q_past = iq_past - iq_ref_past;


s_d = err_d - lamd * err_d_past;
s_q = err_q - lamq * err_q_past;

ud_eq = R*id - Lq*we*iq +(Ld/Tc)*(lamd -1)*id;
ud_n = single(0);

if abs(s_d) > rd*Tc
    ud_n = (ad*(Ld/Tc))*(abs(s_d) - (rd*Tc));
else if abs(s_d) <= rd*Tc
        ud_n = single(0);
end
end

uq_eq = R*iq + Ld*we*id + we*lam0 + (Lq/Tc)*err_q*(lamq - 1);


if abs(s_q)>rq*Tc
    uq_n = (aq*(Lq/Tc))*(abs(s_q) - (rq*Tc));
else
    uq_n = single(0);
end

ud = ud_eq + ud_n;
uq = uq_eq + uq_n;
